simulink model "Pr1model"  (R2017a)
settings: Solver=VariableStepAuto  StartTime=0.0  StopTime=10.0  RelTol=1e-3
libraries: DigiConLib x3
settings Model: Creator=Danny  LastModifiedBy=Danny

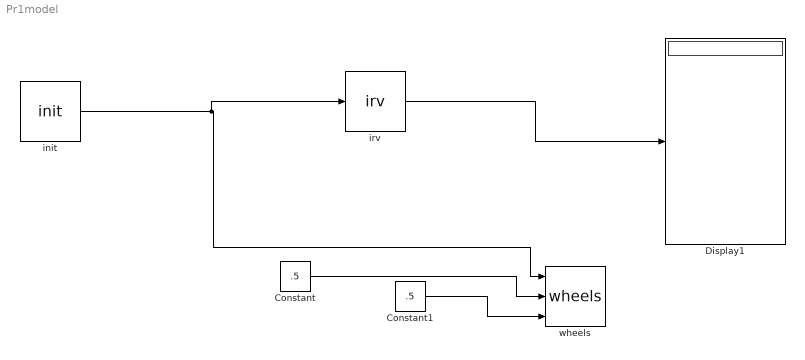
== system Pr1model ==
  Constant : Constant  Value=.5
  Constant1 : Constant  Value=.5
  Display1 : Display
  init : DigiConLib/init
  irv : DigiConLib/irv
  wheels : DigiConLib/wheels
  wires:
  Constant1/1 -> wheels/3
  Constant/1 -> wheels/2
  irv/1 -> Display1/1
  init/1 -> irv/1, wheels/1
